simulink model "untitled"  (R2024a)
settings: Solver=VariableStepAuto  StartTime=0.0  StopTime=10.0  RelTol=1e-3
libraries: mpclib x1
settings Model: Creator=admin  LastModifiedBy=admin

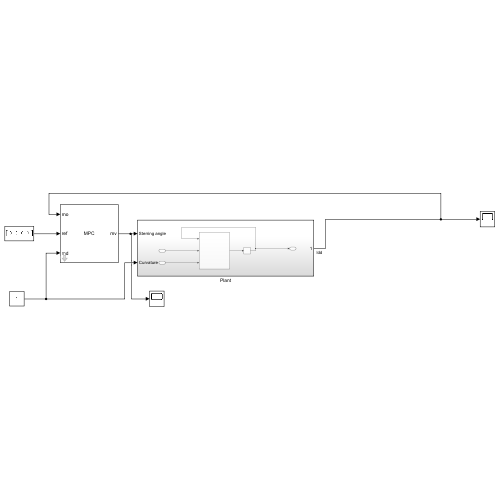
[thumbnail: Simulink's stored preview of the top-level diagram]
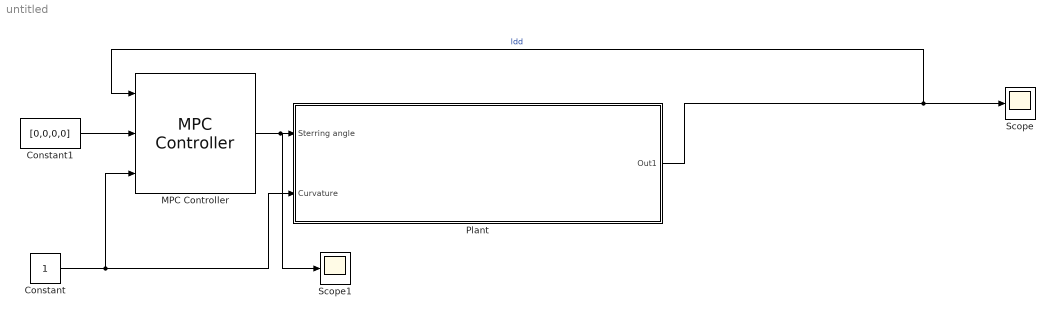
== system untitled ==
  Constant : Constant
  Constant1 : Constant  Value=[0,0,0,0]
  MPC Controller : mpclib/MPC Controller  SCDEnableBlockLinearizationSpecification=on  mpcobj=mpc1  is_multiple=0  enable_value=0  return_u0=off  updateMPCinCallerWorkspace=on  md_inport=on  mv_inport=off  uref_inport=off  return_cost=off  return_mvseq=off  return_qpstatus=off  return_xseq=off  return_state=off  return_ovseq=off  state_inport=off  umin_inport=off  umax_inport=off  ymin_inport=off  ymax_inport=off  cc_inport=off  ywt_inport=off  uwt_inport=off  duwt_inport=off  rhoeps_inport=off  pm_inport=off  MaximumP=10  HorizonChoice=FixedHorizon  n_ts=0.1  n_p=10  n_mv=1  n_md=1  n_ud=0  n_mo=2  n_uo=0  BlockDataType=double  SampleTimeInherited=off  switch_inport=off
  Plant : Subsystem
  Scope : Scope
  Scope1 : Scope
  wires:
  MPC Controller/1 -> Scope1/1, Plant/1(Sterring angle)
  Plant/1(Out1) -> MPC Controller/1, Scope/1  "ldd"
  Constant/1 -> MPC Controller/3, Plant/2(Curvature)
  Constant1/1 -> MPC Controller/2

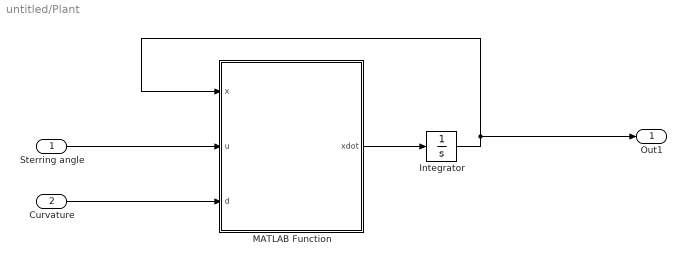
== system untitled/Plant ==
  Sterring angle : Inport
  Curvature : Inport  Port=2
  Integrator : Integrator
  MATLAB Function : MATLAB Function  TreatAsAtomicUnit=on
  Out1 : Outport
  wires:
  Sterring angle/1 -> MATLAB Function/2(u)
  Curvature/1 -> MATLAB Function/3(d)
  MATLAB Function/1(xdot) -> Integrator/1
  Integrator/1 -> MATLAB Function/1(x), Out1/1

== matlab function untitled/Plant/MATLAB Function ==
  data: x input; u input; xdot output; d input
function xdot = laneKeepingModel(x, u, d)
    %#codegen

    % Khởi tạo kích thước đầu ra
    xdot = zeros(4, 1); % Kích thước cố định: vector cột 4x1

    % Các tham số của xe (chọn trước)
    m = 1500;       % Khối lượng xe (kg)
    Iz = 3000;      % Mô men quán tính quanh trục z (kg.m^2)
    Lf = 1.2;       % Khoảng cách từ trọng tâm đến trục bánh trước (m)
    Lr = 1.6;       % Khoảng cách từ trọng tâm đến trục bánh sau (m)
    Caf = 19000;    % Độ cứng góc của bánh trước (N/rad)
    Car = 33000;    % Độ cứng góc của bánh sau (N/rad)
    Vx = 15;        % Vận tốc dọc (m/s)

    % Trạng thái hiện tại
    e1 = x(1);      % Độ lệch ngang
    de1 = x(2);     % Vận tốc lệch ngang
    e2 = x(3);      % Góc lệch yaw
    de2 = x(4);     % Tốc độ quay quanh trục yaw

    % Ma trận trạng thái
    A = [0, 1, 0, 0;
         0, -(2*Caf + 2*Car) / (m * Vx), 0, -(2*Caf*Lf - 2*Car*Lr) / (m * Vx);
         0, 0, 0, 1;
         0, -(2*Caf*Lf - 2*Car*Lr) / (Iz * Vx), 0, -(2*Caf*Lf^2 + 2*Car*Lr^2) / (Iz * Vx)];

    % Ma trận đầu vào
    B = [0;
         2*Caf / m;
         0;
         2*Caf*Lf / Iz];

    % Ma trận nhiễu đo được
    E = [0;
         -Vx;
         0;
         -(2*Caf*Lf - 2*Car*Lr) / (Iz * Vx)];

    % Tính trạng thái tiếp theo
    xdot = A * x + B * u + E * d*Vx;
end
